simulink model "ModelInvertedPD_Plant"  (R2022b)
settings: Solver=ode45  StartTime=0.0  StopTime=20  RelTol=1e-3  EnableMultiTasking=on
undefined symbols (not defined in the file): magnitude
settings Model: Creator=hp  LastModifiedBy=hp
settings SolverCC: AlgebraicLoopSolver=TrustRegion
settings DataIOCC: LimitDataPoints=on  SaveFormat=Array  SignalLoggingSaveFormat=ModelDataLogs  ReturnWorkspaceOutputs=off
settings OptimizationCC: InitFltsAndDblsToZero=on  LifeSpan=inf
settings DebuggingCC: SaveWithParameterizedLinksMsg=none  UnderspecifiedInitializationDetection=Classic  MergeDetectMultiDrivingBlocksExec=none  SignalResolutionControl=TryResolveAllWithWarning  SolverPrmCheckMsg=warning  MultiTaskDSMMsg=warning  MultiTaskCondExecSysMsg=none  FcnCallInpInsideContextMsg=warning  UnconnectedInputMsg=warning  UnconnectedOutputMsg=warning  UnconnectedLineMsg=warning  SFUnexpectedBacktrackingDiag=warning  SFNoUnconditionalDefaultTransitionDiag=warning  SFExecutionAtInitializationDiag=none  SFMachineParentedDataDiag=warning  ArithmeticOperatorsInVariantConditions=warning
settings HardwareCC: ProdBitPerPointer=32  ProdBitPerSizeT=32  ProdBitPerPtrDiffT=32  ProdLargestAtomicFloat=None  ProdIntDivRoundTo=Undefined  ProdEndianess=Unspecified  ProdWordSize=32  ProdHWDeviceType=32-bit Generic
settings ModelReferenceCC: PropagateSignalLabelsOutOfModel=off
settings CodeAppCC: StateflowObjectComments=on
settings GRTTargetCC: TargetFcnLib=ansi_tfl_tmw.mat  TargetLangStandard=C89/C90 (ANSI)  CombineOutputUpdateFcns=off  GRTInterface=on
settings ConfigComp: CovMetricSettings=dw  CovSaveCumulativeToWorkspaceVar=on  CovSaveSingleToWorkspaceVar=on

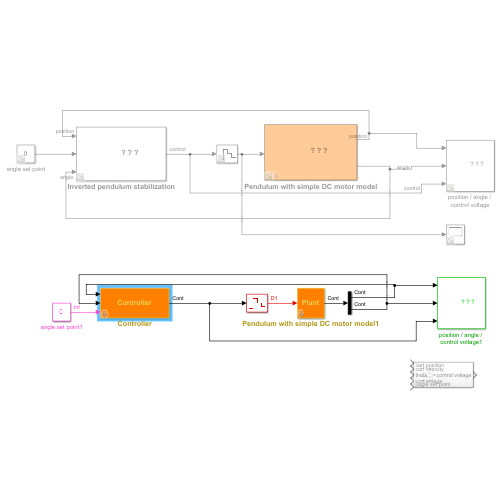
[thumbnail: Simulink's stored preview of the top-level diagram]
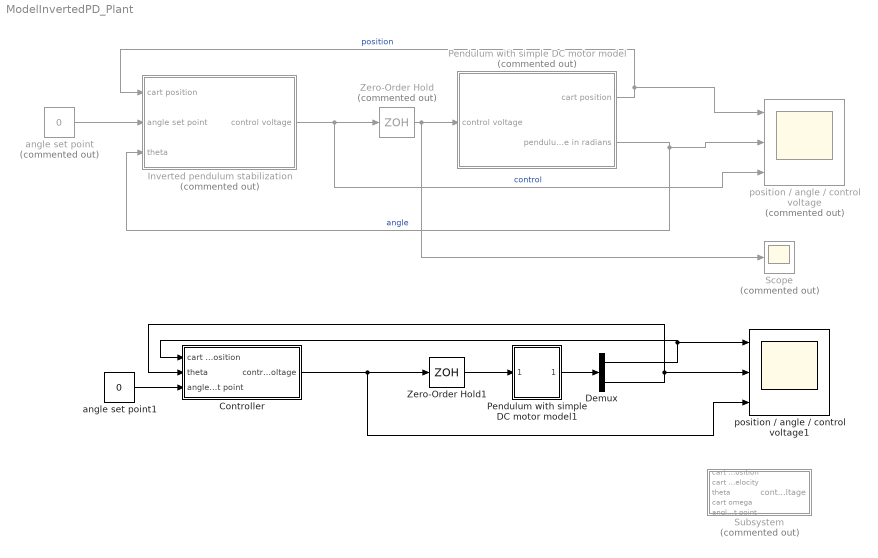
== system ModelInvertedPD_Plant ==
  Controller : Subsystem  mask{m=0.23, cM=2.4, L=0.4, g=9.81, I=0.099, theta0=0.2, cart_friction=0.05, pend_damp=0.005}
      mask prompts: m "Pendulum mass"; cM "Cart mass"; L "Pendulum length"; g "gravitational constant"; I "Moment of inertia of the pole itself"; theta0 "Initial pendulum angle"; cart_friction "Cart friction coefficient"; pend_damp "Pendulum damping coefficient"
      mask Display: fprintf("Controller");
  Demux : Demux  Outputs=2
  Inverted pendulum stabilization : Subsystem  Commented=on
      mask Display: image(imread('bckg.bmp'))disp('Inverted pendulum \nstabilization')
  Pendulum with simple DC motor model : Subsystem  Commented=on  mask{m=0.23, cM=2.4, L=0.4, g=9.81, I=0.099, theta0=0.2, cart_friction=0.05, pend_damp=0.005}
      mask prompts: m "Pendulum mass"; cM "Cart mass"; L "Pendulum length"; g "gravitational constant"; I "Moment of inertia of the pole itself"; theta0 "Initial pendulum angle"; cart_friction "Cart friction coefficient"; pend_damp "Pendulum damping coefficient"
      mask Display: image(imread('pend.bmp'))
  Pendulum with simple DC motor model1 : Subsystem  mask{m=0.23, cM=2.4, L=0.4, g=9.81, I=0.099, theta0=0.2, cart_friction=0.05, pend_damp=0.005}
      mask prompts: m "Pendulum mass"; cM "Cart mass"; L "Pendulum length"; g "gravitational constant"; I "Moment of inertia of the pole itself"; theta0 "Initial pendulum angle"; cart_friction "Cart friction coefficient"; pend_damp "Pendulum damping coefficient"
      mask Display: fprintf("Plant");
  Scope : Scope  Commented=on
  Subsystem : Subsystem  Commented=on
  Zero-Order Hold : ZeroOrderHold  Commented=on  SampleTime=0.001
  Zero-Order Hold1 : ZeroOrderHold  SampleTime=0.001
  angle set point : Constant  Commented=on  Value=0
  angle set point1 : Constant  Value=0  VectorParams1D=off
  position / angle / control voltage : Scope  Commented=on  NumInputPorts=3
      mask Display: image(imread('scope.jpg'))
  position / angle / control voltage1 : Scope  NumInputPorts=3
      mask Display: image(imread('scope.jpg'))
  wires:
  Pendulum with simple DC motor model/1(cart position) -> Inverted pendulum stabilization/1(cart position), position / angle / control voltage/1  "position"
  Pendulum with simple DC motor model/2(pendulum angle in radians) -> Inverted pendulum stabilization/3(theta), position / angle / control voltage/2  "angle"
  angle set point/1 -> Inverted pendulum stabilization/2(angle set point)
  Inverted pendulum stabilization/1(control voltage) -> Zero-Order Hold/1, position / angle / control voltage/3  "control"
  Zero-Order Hold/1 -> Scope/1, Pendulum with simple DC motor model/1(control voltage)
  Zero-Order Hold1/1 -> Pendulum with simple DC motor model1/1(control voltage)
  angle set point1/1 -> Controller/3(angle set point)
  Pendulum with simple DC motor model1/1(state) -> Demux/1
  Controller/1(control voltage) -> position / angle / control voltage1/3, Zero-Order Hold1/1
  Demux/1 -> Controller/1(cart position), position / angle / control voltage1/1
  Demux/2 -> Controller/2(theta), position / angle / control voltage1/2

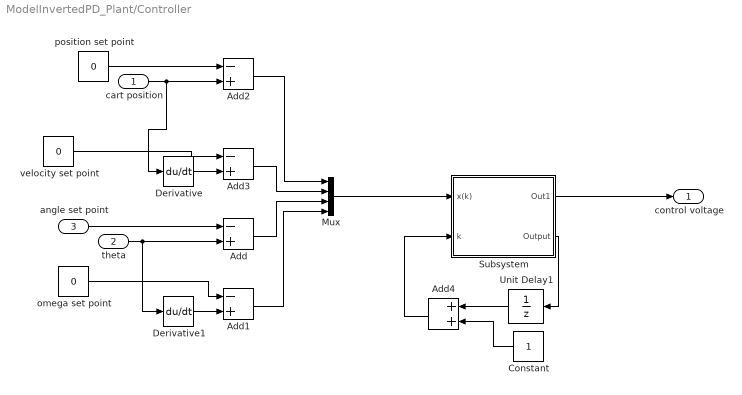
== system ModelInvertedPD_Plant/Controller ==
  cart position : Inport
  theta : Inport  Port=2
  angle set point : Inport  Port=3
  Add{,1..3} (4 alike) : Sum  Inputs=-+
  Add4 : Sum
  Constant : Constant
  Derivative : Derivative
  Derivative1 : Derivative
  Mux : Mux
  Subsystem : Subsystem  mask{ao=0.1, e=10, ko=2, tf=9, A=|, B=|, C=[-0.0408, -0.3333 ,0,  0.1228];}
      mask A=|
      | [0      1              0           0;
      |      0 -(I+m*l^2)*b/p  -(m^2*g*l^2)/p   +m*l*k/p;
      |      0      0              0           1;
      |      0 +(m*l*b)/p       m*g*l*(M+m)/p -k*(M+m)/p];
      mask B=|
      | [     0;
      |      (I+m*l^2)/p;
      |           0;
      |         -m*l/p];
  Unit Delay1 : UnitDelay  InitialCondition=1  SampleTime=-1  HasFrameUpgradeWarning=on
  omega set point : Constant  Value=0
  position set point : Constant  Value=0
  velocity set point : Constant  Value=0
  control voltage : Outport
  wires:
  Add1/1 -> Mux/4
  Add2/1 -> Mux/1
  Add3/1 -> Mux/2
  Add/1 -> Mux/3
  position set point/1 -> Add2/1
  velocity set point/1 -> Add3/1
  omega set point/1 -> Add1/1
  angle set point/1 -> Add/1
  Mux/1 -> Subsystem/1(x(k))
  Subsystem/1(Out1) -> control voltage/1
  Subsystem/2(Output) -> Unit Delay1/1
  Unit Delay1/1 -> Add4/1
  Constant/1 -> Add4/2
  Add4/1 -> Subsystem/2(k)
  Derivative/1 -> Add3/2
  theta/1 -> Derivative1/1, Add/2
  cart position/1 -> Derivative/1, Add2/2
  Derivative1/1 -> Add1/2

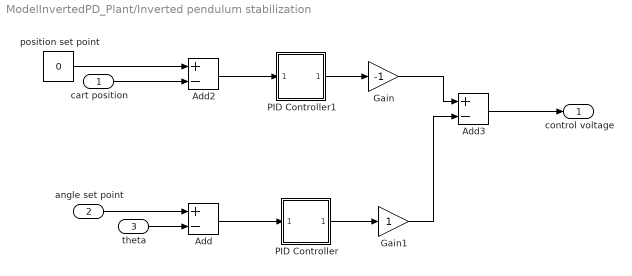
== system ModelInvertedPD_Plant/Inverted pendulum stabilization ==
  cart position : Inport
  angle set point : Inport  Port=2
  theta : Inport  Port=3
  Add : Sum  Inputs=+-
  Add2 : Sum  Inputs=+-
  Add3 : Sum  Inputs=+-
  Gain : Gain  Gain=-1
  Gain1 : Gain
  PID Controller : Subsystem  AncestorBlock=simulink_extras/Additional Linear/PID Controller  mask(PID Controller){P=40, I=5, D=9}
      mask prompts: P "Proportional:"; I "Integral:"; D "Derivative:"
      mask help:
      | Enter expressions for proportional, integral, and derivative terms.
      | P+I/s+Ds
      settings: LibrarySourceBlock=|
      | simulink_extras/Additional
      | Linear/PID Controller
      mask Help: This block implements a PID controller where parameters are entered for the Proportional, Integral and Derivative terms. Unmask this block to see how it works. The derivative term is implemented using a true derivative block.
      mask Display: image(imread('bckg.bmp'))disp('PID')
  PID Controller1 : Subsystem  AncestorBlock=simulink_extras/Additional Linear/PID Controller  mask(PID Controller){P=0.2, I=0.001, D=0}
      mask prompts: P "Proportional:"; I "Integral:"; D "Derivative:"
      mask help:
      | Enter expressions for proportional, integral, and derivative terms.
      | P+I/s+Ds
      settings: LibrarySourceBlock=|
      | simulink_extras/Additional
      | Linear/PID Controller
      mask Help: This block implements a PID controller where parameters are entered for the Proportional, Integral and Derivative terms. Unmask this block to see how it works. The derivative term is implemented using a true derivative block.
      mask Display: image(imread('bckg.bmp'))disp('PID')
  position set point : Constant  Value=0
  control voltage : Outport
  wires:
  PID Controller/1(Out_1) -> Gain1/1
  Add/1 -> PID Controller/1(In_1)
  position set point/1 -> Add2/1
  Add2/1 -> PID Controller1/1(In_1)
  PID Controller1/1(Out_1) -> Gain/1
  Gain/1 -> Add3/1
  cart position/1 -> Add2/2
  theta/1 -> Add/2
  angle set point/1 -> Add/1
  Add3/1 -> control voltage/1
  Gain1/1 -> Add3/2

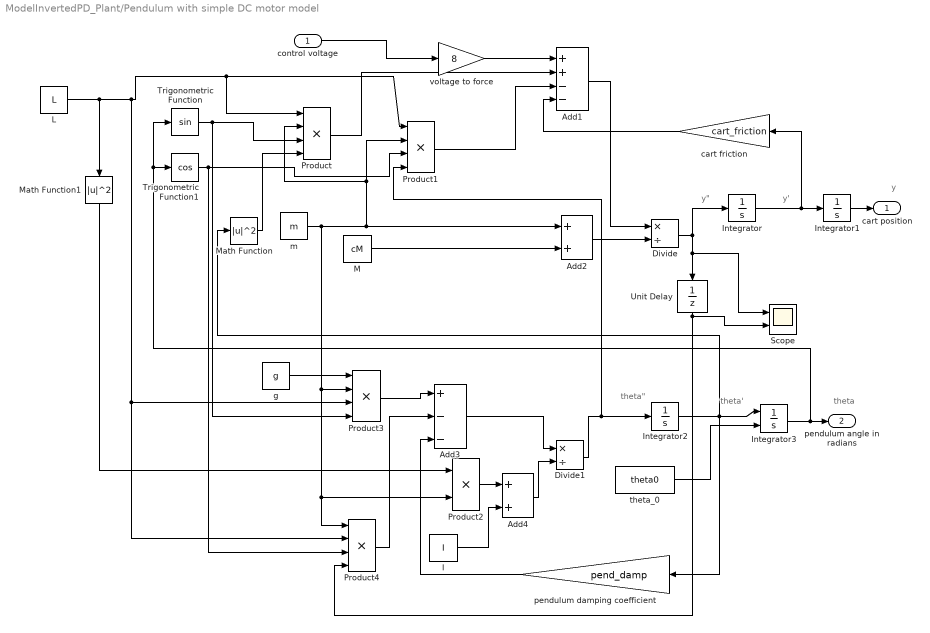
== system ModelInvertedPD_Plant/Pendulum with simple DC motor model ==
  note: y"
  note: y'
  note: theta"
  note: theta'
  note: theta
  note: y
  control voltage : Inport
  Add1 : Sum  Inputs=++--
  Add2 : Sum
  Add3 : Sum  Inputs=+--
  Add4 : Sum
  Divide : Product  Inputs=*/
  Divide1 : Product  Inputs=*/
  I : Constant  Value=I
  Integrator : Integrator
  Integrator1 : Integrator
  Integrator2 : Integrator
  Integrator3 : Integrator  InitialConditionSource=external
  L : Constant  Value=L
  M : Constant  Value=cM
  Math Function : Math  Operator=magnitude^2  SignedPower=on
  Math Function1 : Math  Operator=magnitude^2  SignedPower=on
  Product{,1,3..4} (4 alike) : Product  Inputs=4  RndMeth=Zero
  Product2 : Product  RndMeth=Zero
  Scope : Scope  NumInputPorts=2
  Trigonometric Function : Trigonometry
  Trigonometric Function1 : Trigonometry  Operator=cos
  Unit Delay : UnitDelay  SampleTime=0.001
  cart friction : Gain  Gain=cart_friction
  g : Constant  Value=g
  m : Constant  Value=m
  pendulum damping coefficient : Gain  Gain=pend_damp
  theta_0 : Constant  Value=theta0
  voltage to force : Gain  Gain=8
  cart position : Outport
  pendulum angle in radians : Outport  Port=2
  wires:
  Unit Delay/1 -> Scope/2, Product4/4
  voltage to force/1 -> Add1/1
  I/1 -> Add4/2
  Add4/1 -> Divide1/2
  Product2/1 -> Add4/1
  Integrator1/1 -> cart position/1
  control voltage/1 -> voltage to force/1
  pendulum damping coefficient/1 -> Add3/3
  cart friction/1 -> Add1/4
  g/1 -> Product3/1
  Product4/1 -> Add3/2
  Product3/1 -> Add3/1
  Math Function1/1 -> Product2/1
  Add3/1 -> Divide1/1
  Trigonometric Function1/1 -> Product4/3, Product1/3
  Product1/1 -> Add1/3
  Product/1 -> Add1/2
  Math Function/1 -> Product/4
  theta_0/1 -> Integrator3/2
  Trigonometric Function/1 -> Product3/4, Product/3
  L/1 -> Product4/2, Product3/3, Product1/1, Product/1, Math Function1/1
  Divide1/1 -> Product1/4, Integrator2/1
  Divide/1 -> Scope/1, Unit Delay/1, Integrator/1
  Add1/1 -> Divide/1
  Add2/1 -> Divide/2
  M/1 -> Add2/2
  m/1 -> Product4/1, Product2/2, Product3/2, Product1/2, Product/2, Add2/1
  Integrator3/1 -> pendulum angle in radians/1, Trigonometric Function/1, Trigonometric Function1/1
  Integrator2/1 -> pendulum damping coefficient/1, Math Function/1, Integrator3/1
  Integrator/1 -> cart friction/1, Integrator1/1

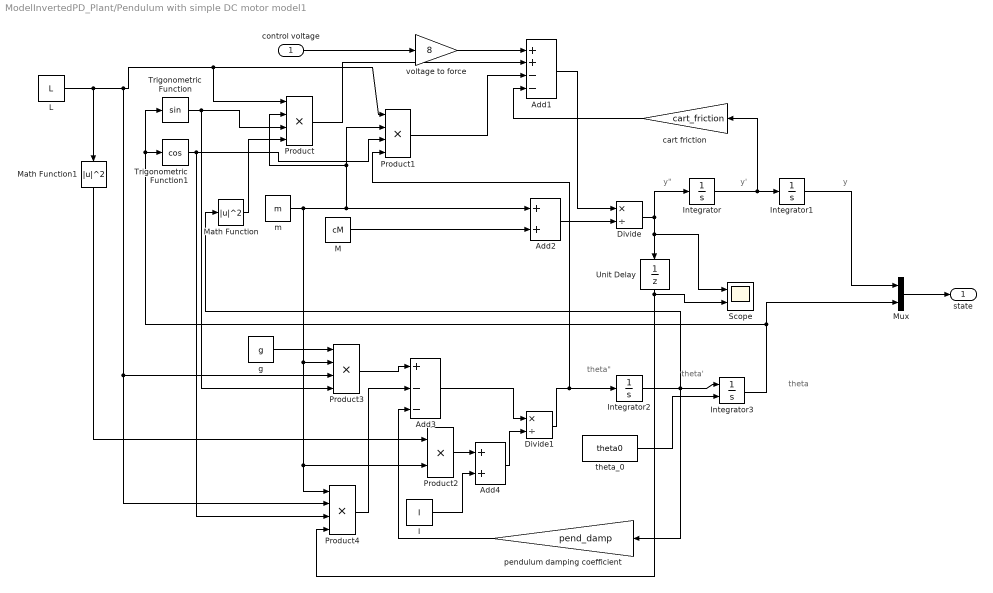
== system ModelInvertedPD_Plant/Pendulum with simple DC motor model1 ==
  note: y
  note: theta
  note: theta'
  note: theta"
  note: y'
  note: y"
  control voltage : Inport
  Add1 : Sum  Inputs=++--
  Add2 : Sum
  Add3 : Sum  Inputs=+--
  Add4 : Sum
  Divide : Product  Inputs=*/
  Divide1 : Product  Inputs=*/
  I : Constant  Value=I
  Integrator : Integrator
  Integrator1 : Integrator
  Integrator2 : Integrator
  Integrator3 : Integrator  InitialConditionSource=external
  L : Constant  Value=L
  M : Constant  Value=cM
  Math Function : Math  Operator=magnitude^2  SignedPower=on
  Math Function1 : Math  Operator=magnitude^2  SignedPower=on
  Mux : Mux  Inputs=2
  Product{,1,3..4} (4 alike) : Product  Inputs=4  RndMeth=Zero
  Product2 : Product  RndMeth=Zero
  Scope : Scope  NumInputPorts=2
  Trigonometric Function : Trigonometry
  Trigonometric Function1 : Trigonometry  Operator=cos
  Unit Delay : UnitDelay  SampleTime=0.001
  cart friction : Gain  Gain=cart_friction
  g : Constant  Value=g
  m : Constant  Value=m
  pendulum damping coefficient : Gain  Gain=pend_damp
  theta_0 : Constant  Value=theta0
  voltage to force : Gain  Gain=8
  state : Outport
  wires:
  Integrator/1 -> Integrator1/1, cart friction/1
  Integrator2/1 -> Integrator3/1, Math Function/1, pendulum damping coefficient/1
  Integrator3/1 -> Mux/2, Trigonometric Function1/1, Trigonometric Function/1
  m/1 -> Add2/1, Product/2, Product1/2, Product3/2, Product2/2, Product4/1
  M/1 -> Add2/2
  Add2/1 -> Divide/2
  Add1/1 -> Divide/1
  Divide/1 -> Integrator/1, Unit Delay/1, Scope/1
  Divide1/1 -> Integrator2/1, Product1/4
  L/1 -> Math Function1/1, Product/1, Product1/1, Product3/3, Product4/2
  Trigonometric Function/1 -> Product/3, Product3/4
  theta_0/1 -> Integrator3/2
  Math Function/1 -> Product/4
  Product/1 -> Add1/2
  Product1/1 -> Add1/3
  Trigonometric Function1/1 -> Product1/3, Product4/3
  Add3/1 -> Divide1/1
  Math Function1/1 -> Product2/1
  Product3/1 -> Add3/1
  Product4/1 -> Add3/2
  g/1 -> Product3/1
  cart friction/1 -> Add1/4
  pendulum damping coefficient/1 -> Add3/3
  control voltage/1 -> voltage to force/1
  Product2/1 -> Add4/1
  Add4/1 -> Divide1/2
  I/1 -> Add4/2
  voltage to force/1 -> Add1/1
  Unit Delay/1 -> Product4/4, Scope/2
  Integrator1/1 -> Mux/1
  Mux/1 -> state/1

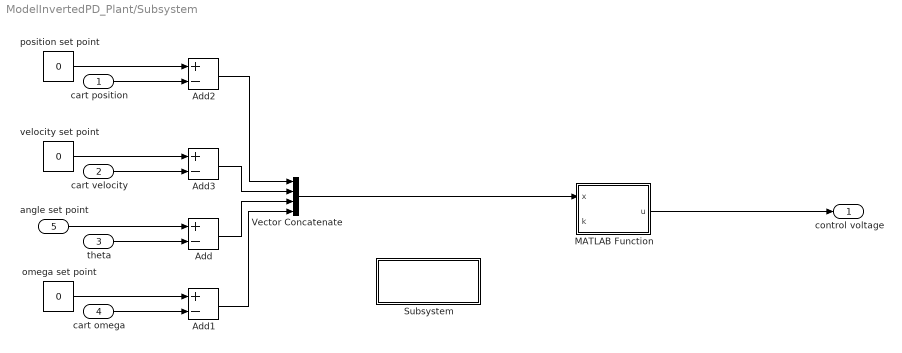
== system ModelInvertedPD_Plant/Subsystem ==
  cart position : Inport
  cart velocity : Inport  Port=2
  theta : Inport  Port=3
  cart omega : Inport  Port=4
  angle set point : Inport  Port=5
  Add{,1..3} (4 alike) : Sum  Inputs=+-
  MATLAB Function : MATLAB Function  TreatAsAtomicUnit=on
  Subsystem : Subsystem  mask{e=0, k=0, coefficient_friction=0, A=double, B=double}
  Vector Concatenate : Concatenate  NumInputs=4
  omega set point : Constant  Value=0
  position set point : Constant  Value=0
  velocity set point : Constant  Value=0
  control voltage : Outport
  wires:
  cart position/1 -> Add2/2
  position set point/1 -> Add2/1
  theta/1 -> Add/2
  MATLAB Function/1(u) -> control voltage/1
  angle set point/1 -> Add/1
  Vector Concatenate/1 -> MATLAB Function/1(x)
  cart omega/1 -> Add1/2
  cart velocity/1 -> Add3/2
  velocity set point/1 -> Add3/1
  omega set point/1 -> Add1/1
  Add2/1 -> Vector Concatenate/1
  Add3/1 -> Vector Concatenate/2
  Add/1 -> Vector Concatenate/3
  Add1/1 -> Vector Concatenate/4

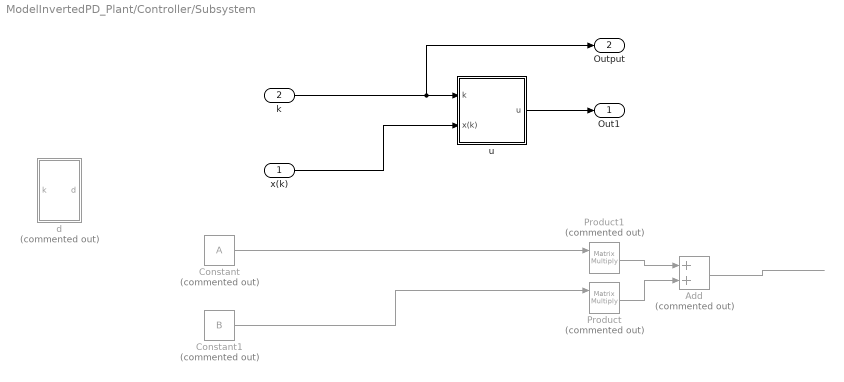
== system ModelInvertedPD_Plant/Controller/Subsystem ==
  x(k) : Inport
  k : Inport  Port=2
  Add : Sum  Commented=on
  Constant : Constant  Commented=on  Value=A
  Constant1 : Constant  Commented=on  Value=B  VectorParams1D=off
  Product : Product  Commented=on  Multiplication=Matrix(*)
  Product1 : Product  Commented=on  Multiplication=Matrix(*)
  d : Subsystem  Commented=on
  u : Subsystem
  Out1 : Outport
  Output : Outport  Port=2
  wires:
  k/1 -> Output/1, u/1(k)
  x(k)/1 -> u/2(x(k))
  u/1(u) -> Out1/1
  Constant1/1 -> Product/1
  Constant/1 -> Product1/1
  Product1/1 -> Add/1
  Product/1 -> Add/2
  Add/1 -> ?

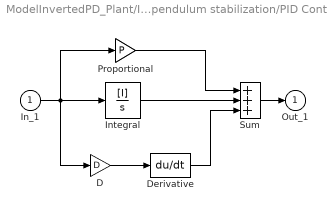
== system ModelInvertedPD_Plant/Inverted pendulum stabilization/PID Controller ==
  In_1 : Inport
  D : Gain  Gain=D  SaturateOnIntegerOverflow=on  OutDataTypeStr=Inherit: Same as input  ParamDataTypeStr=Inherit: Same as input
  Derivative : Derivative
  Integral : TransferFcn  Numerator=[I]  Denominator=[1 0]
  Proportional : Gain  Gain=P  SaturateOnIntegerOverflow=on  OutDataTypeStr=Inherit: Same as input  ParamDataTypeStr=Inherit: Same as input
  Sum : Sum  Inputs=+++  InputSameDT=on  SaturateOnIntegerOverflow=on  OutDataTypeStr=Inherit: Same as first input
  Out_1 : Outport  InitialOutput=0
  wires:
  Proportional/1 -> Sum/1
  Integral/1 -> Sum/2
  Derivative/1 -> Sum/3
  In_1/1 -> Integral/1, Proportional/1, D/1
  Sum/1 -> Out_1/1
  D/1 -> Derivative/1

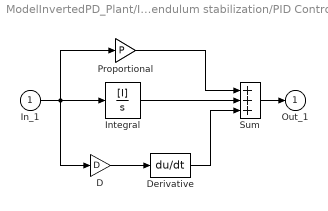
== system ModelInvertedPD_Plant/Inverted pendulum stabilization/PID Controller1 ==
  In_1 : Inport
  D : Gain  Gain=D  SaturateOnIntegerOverflow=on  OutDataTypeStr=Inherit: Same as input  ParamDataTypeStr=Inherit: Same as input
  Derivative : Derivative
  Integral : TransferFcn  Numerator=[I]  Denominator=[1 0]
  Proportional : Gain  Gain=P  SaturateOnIntegerOverflow=on  OutDataTypeStr=Inherit: Same as input  ParamDataTypeStr=Inherit: Same as input
  Sum : Sum  Inputs=+++  InputSameDT=on  SaturateOnIntegerOverflow=on  OutDataTypeStr=Inherit: Same as first input
  Out_1 : Outport  InitialOutput=0
  wires:
  Proportional/1 -> Sum/1
  Integral/1 -> Sum/2
  Derivative/1 -> Sum/3
  In_1/1 -> Integral/1, Proportional/1, D/1
  Sum/1 -> Out_1/1
  D/1 -> Derivative/1

== system ModelInvertedPD_Plant/Subsystem/Subsystem ==

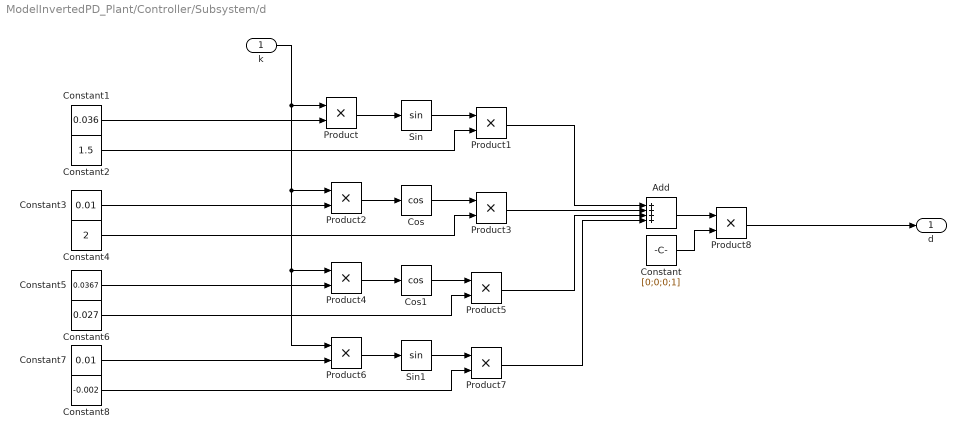
== system ModelInvertedPD_Plant/Controller/Subsystem/d ==
  k : Inport
  Add : Sum  Inputs=++++
  Constant : Constant  Value=[0;0;0;1]  VectorParams1D=off
  Constant1 : Constant  Value=0.036
  Constant2 : Constant  Value=1.5
  Constant3 : Constant  Value=0.01
  Constant4 : Constant  Value=2
  Constant5 : Constant  Value=0.0367
  Constant6 : Constant  Value=0.027
  Constant7 : Constant  Value=0.01
  Constant8 : Constant  Value=-0.002
  Cos : Trigonometry  Operator=cos
  Cos1 : Trigonometry  Operator=cos
  Product{,1..8} (9 alike) : Product
  Sin : Trigonometry
  Sin1 : Trigonometry
  d : Outport
  wires:
  Cos/1 -> Product3/1
  Constant8/1 -> Product7/2
  Sin1/1 -> Product7/1
  Cos1/1 -> Product5/1
  Product2/1 -> Cos/1
  Constant7/1 -> Product6/2
  Sin/1 -> Product1/1
  Product/1 -> Sin/1
  k/1 -> Product6/1, Product4/1, Product2/1, Product/1
  Product8/1 -> d/1
  Constant4/1 -> Product3/2
  Product3/1 -> Add/2
  Add/1 -> Product8/1
  Constant1/1 -> Product/2
  Product7/1 -> Add/4
  Constant3/1 -> Product2/2
  Constant5/1 -> Product4/2
  Constant6/1 -> Product5/2
  Product5/1 -> Add/3
  Product4/1 -> Cos1/1
  Constant2/1 -> Product1/2
  Constant/1 -> Product8/2
  Product6/1 -> Sin1/1
  Product1/1 -> Add/1

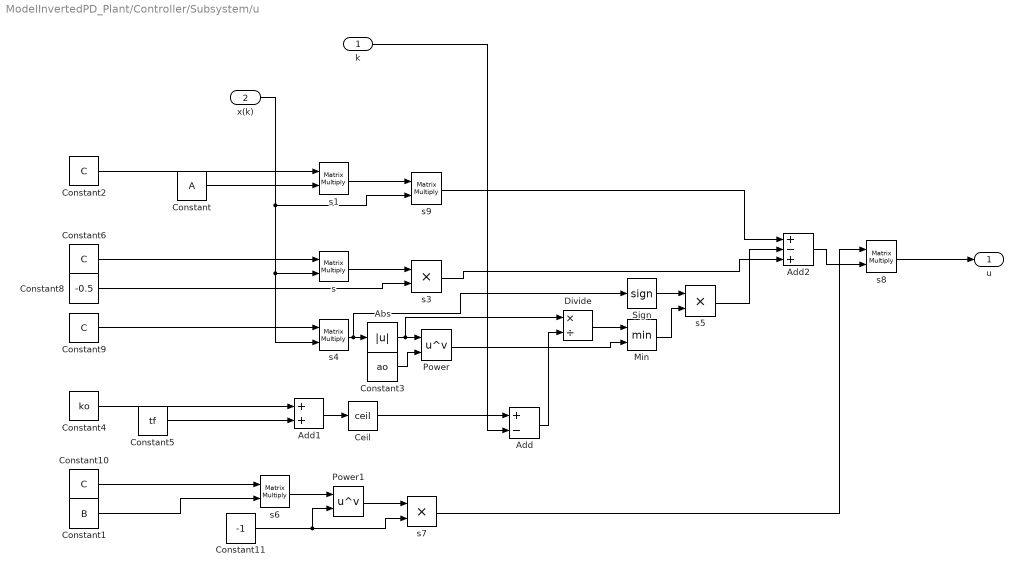
== system ModelInvertedPD_Plant/Controller/Subsystem/u ==
  k : Inport  PortDimensions=1
  x(k) : Inport  Port=2  PortDimensions=[4 1]
  Abs : Abs  SaturateOnIntegerOverflow=off
  Add : Sum  Inputs=+-
  Add1 : Sum
  Add2 : Sum  Inputs=+-+
  Ceil : Rounding  Operator=ceil
  Constant : Constant  Value=A  VectorParams1D=off
  Constant1 : Constant  Value=B  VectorParams1D=off
  Constant{2,6,9..10} (4 alike) : Constant  Value=C  VectorParams1D=off
  Constant11 : Constant  Value=-1
  Constant3 : Constant  Value=ao
  Constant4 : Constant  Value=ko
  Constant5 : Constant  Value=tf
  Constant8 : Constant  Value=-0.5  VectorParams1D=off
  Divide : Product  Inputs=*/
  Min : MinMax  Inputs=2
  Power : Math  Operator=pow
  Power1 : Math  Operator=pow
  Sign : Signum
  s{,1,4,6,8..9} (6 alike) : Product  Multiplication=Matrix(*)
  s3 : Product
  s5 : Product
  s7 : Product
  u : Outport
  wires:
  s8/1 -> u/1
  Constant/1 -> s1/2
  Sign/1 -> s5/1
  Constant8/1 -> s3/2
  s/1 -> s3/1
  Constant6/1 -> s/1
  s5/1 -> Add2/2
  Constant9/1 -> s4/1
  Add1/1 -> Ceil/1
  x(k)/1 -> s4/2, s/2, s9/2
  s4/1 -> Sign/1, Abs/1
  s3/1 -> Add2/3
  s6/1 -> Power1/1
  Ceil/1 -> Add/1
  Add2/1 -> s8/2
  s7/1 -> s8/1
  Divide/1 -> Min/1
  Constant4/1 -> Add1/1
  Add/1 -> Divide/2
  Power1/1 -> s7/1
  Min/1 -> s5/2
  Constant11/1 -> s7/2, Power1/2
  Abs/1 -> Divide/1, Power/1
  Constant2/1 -> s1/1
  Constant10/1 -> s6/1
  Constant1/1 -> s6/2
  Constant3/1 -> Power/2
  Constant5/1 -> Add1/2
  Power/1 -> Min/2
  k/1 -> Add/2
  s1/1 -> s9/1
  s9/1 -> Add2/1

== matlab function ModelInvertedPD_Plant/Subsystem/MATLAB Function ==
  data: x input; u output; k input
function u = fcn(x,k)
M = 2.4;
m = 0.23;
b = 0.05;
I = 0.099;
g = 9.81;
l = 0.4;
% constants
a=.1;
e = 10;
ko = 2;
tf = 9;

p = I*(M+m)+M*m*l^2; %denominator for the A and B matrices

A = [0      1              0           0;
     0 -(I+m*l^2)*b/p  (m^2*g*l^2)/p   -m*l*k/p;
     0      0              0           1;
     0 -(m*l*b)/p       m*g*l*(M+m)/p  k*(M+m)/p];
B = [     0;
     (I+m*l^2)/p;
          0;
        m*l/p];
C = [2.9659 0.6724 6.8462 1];

s = C*x;
d = [0; 0; 0; 1]*(1.5*sin(0.036*k)+2*cos(0.01*k)+0.027*cos(0.0367*k)-0.002*sin(0.01*k));
u = -(C*B)^-1*[C*A*x + C*d - 0.5*s - sign(s)*min((abs(s))^a,(abs(s)/(ceil(tf+ko)-k)))];
